simulink model "P1"  (R2025b)
settings: Solver=VariableStepAuto  StartTime=0.0  StopTime=10.0  RelTol=1e-3
values from neighbouring files (symbols this model uses):
  alpha_0 = deg2rad(1)    [PR1.m]
  Beq = 0.25    [PR1.m]
  Bp = 0.2    [PR1.m]
  d_alpha_0 = 0    [PR1.m]
  d_xc_0 = 0    [PR1.m]
  Fc = 0    [PR.m]    (also in PR1.m = 0.2)
  g = 9.81    [PR1.m]
  Ip = 0.2    [PR1.m]
  lp = 0.3    [PR1.m]
  Mc = 0.2    [PR1.m]
  Mp = 0.1    [PR1.m]
  xc_0 = 0    [PR1.m]
settings Model: Creator=juani  LastModifiedBy=juani

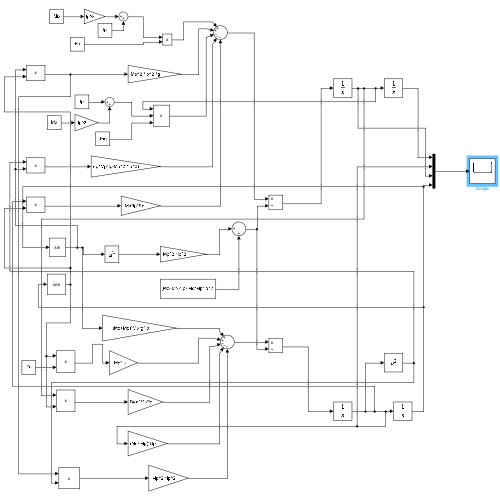
[thumbnail: Simulink's stored preview of the top-level diagram]
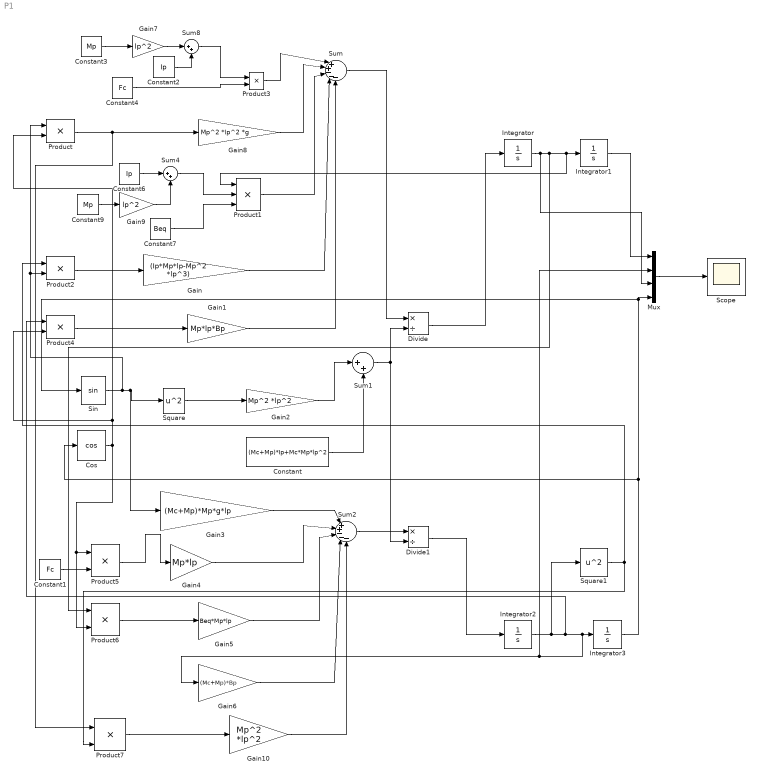
== system P1 ==
  Constant : Constant  Value=(Mc+Mp)*Ip+Mc*Mp*lp^2
  Constant1 : Constant  Value=Fc
  Constant2 : Constant  Value=Ip
  Constant3 : Constant  Value=Mp
  Constant4 : Constant  Value=Fc
  Constant6 : Constant  Value=Ip
  Constant7 : Constant  Value=Beq
  Constant9 : Constant  Value=Mp
  Cos : Trigonometry  Operator=cos
  Divide : Product  Inputs=*/
  Divide1 : Product  Inputs=*/
  Gain : Gain  Gain=(Ip*Mp*lp-Mp^2 *lp^3)
  Gain1 : Gain  Gain=Mp*lp*Bp
  Gain10 : Gain  Gain=Mp^2 *lp^2
  Gain2 : Gain  Gain=Mp^2 *lp^2
  Gain3 : Gain  Gain=(Mc+Mp)*Mp*g*lp
  Gain4 : Gain  Gain=Mp*lp
  Gain5 : Gain  Gain=Beq*Mp*lp
  Gain6 : Gain  Gain=(Mc+Mp)*Bp
  Gain7 : Gain  Gain=lp^2
  Gain8 : Gain  Gain=Mp^2 *lp^2 *g
  Gain9 : Gain  Gain=lp^2
  Integrator : Integrator  InitialCondition=xc_0
  Integrator1 : Integrator  InitialCondition=d_xc_0
  Integrator2 : Integrator  InitialCondition=alpha_0
  Integrator3 : Integrator  InitialCondition=d_alpha_0
  Mux : Mux
  Product{,2..7} (7 alike) : Product
  Product1 : Product  Inputs=3
  Scope : Scope
      settings: ActiveDisplayYMinimum=-12.404521830000444  ActiveDisplayYMaximum=104.30183744023992
  Sin : Trigonometry
  Square : Math  Operator=square
  Square1 : Math  Operator=square
  Sum : Sum  Inputs=|++---
  Sum1 : Sum  Inputs=|++
  Sum2 : Sum  Inputs=|++---
  Sum4 : Sum  Inputs=|++
  Sum8 : Sum  Inputs=|++
  wires:
  Constant2/1 -> Sum8/2
  Gain7/1 -> Sum8/1
  Constant3/1 -> Gain7/1
  Constant4/1 -> Product3/2
  Sum8/1 -> Product3/1
  Product3/1 -> Sum/1
  Product/1 -> Product7/1, Gain8/1
  Gain8/1 -> Sum/2
  Sum4/1 -> Product1/2
  Constant6/1 -> Sum4/1
  Gain9/1 -> Sum4/2
  Constant9/1 -> Gain9/1
  Constant7/1 -> Product1/3
  Product1/1 -> Sum/3
  Product2/1 -> Gain/1
  Gain/1 -> Sum/4
  Gain1/1 -> Sum/5
  Product4/1 -> Gain1/1
  Sum/1 -> Divide/1
  Divide/1 -> Integrator/1
  Integrator/1 -> Mux/3, Product6/1, Product1/1, Integrator1/1
  Integrator1/1 -> Mux/1
  Sin/1 -> Product2/2, Product/1, Gain3/1, Square/1
  Square/1 -> Gain2/1
  Sum1/1 -> Divide1/2, Divide/2
  Gain2/1 -> Sum1/1
  Constant/1 -> Sum1/2
  Cos/1 -> Product6/2, Product5/1, Product4/2, Product/2
  Gain3/1 -> Sum2/1
  Constant1/1 -> Product5/2
  Product5/1 -> Gain4/1
  Gain4/1 -> Sum2/2
  Product6/1 -> Gain5/1
  Gain5/1 -> Sum2/3
  Gain6/1 -> Sum2/4
  Gain10/1 -> Sum2/5
  Product7/1 -> Gain10/1
  Sum2/1 -> Divide1/1
  Integrator2/1 -> Square1/1, Product4/1, Mux/2, Gain6/1, Integrator3/1
  Divide1/1 -> Integrator2/1
  Square1/1 -> Product7/2, Product2/1
  Integrator3/1 -> Cos/1, Sin/1, Mux/4
  Mux/1 -> Scope/1
